simulink model "control_scenario2"  (Simulink 8.9)
settings: Solver=FixedStepAuto  StartTime=0.0  StopTime=20  MaxStep=0.01  RelTol=1e-4  EnableMultiTasking=on
undefined symbols (not defined in the file or in its folder): sigbuilder_block
libraries: fuzblock x1
settings Model: LogicAnalyzerSignalOrdering=6b2a1942-3d28-4729-8a02-0566cc64ad92,33d7c2ba-298a-487f-a15a-bbe0029d2366,768ba1eb-50de-46f7-9be9-bebabd7bf970,4ab0f0e9-8454-41f6-a2d7-33861cd3e8d9  SuppressorTable=22 serialization::archive 11 0 6 0 0 0 11 0  Creator=root  LastModifiedBy=root
settings Model: LogicAnalyzerGraphicalSettings=|
  | {
  |   "cursors" : {
  |     "activeCursor" : 0,
  |     "lockedCursors" : [
  | 
  |     ],
  |     "startingCursor" : 0,
  |     "times" : [
  |       0
  |     ]
  |   },
  |   "global" : {
  |   },
  |   "panels" : [
  |     {
  |       "height" : 100,
  |       "startingTrace" : 0,
  |       "traces" : [
  |         {
  |           "signalId" : "33d7c2ba-298a-487f-a15a-bbe0029d2366",
  |           "type" : "wave"
  |         },
  |         {
  |           "signalId" : "768ba1eb-50de-46f7-9be9-bebabd7bf970",
  |           "type" : "wave"
  |         },
  |         {
  |           "signalId" : "4ab0f0e9-8454-41f6-a2d7-33861cd3e8d9",
  |           "type" : "wave"
  |         },
  |         {
  |           "signalId" : "6b2a1942-3d28-4729-8a02-0566cc64ad92",
  |           "type" : "wave"
  |         }
  |       ],
  |       "yOffset" : 0
  |     }
  |   ],
  |   "timeAxis" : {
  |     "displayUnits" : "",
  |     "pixelsPerSecond" : 293
  |   }
  | }
settings DataIOCC: SaveFormat=Dataset  SignalLoggingSaveFormat=Dataset  SaveOutput=off  SaveTime=off
settings OptimizationCC: ExpressionDepthLimit=2147483647  LifeSpan=1
settings DebuggingCC: AllowSymbolicDim=off
settings HardwareCC: ProdBitPerPointer=64  ProdBitPerSizeT=64  ProdBitPerPtrDiffT=64  ProdLargestAtomicFloat=Float  ProdIntDivRoundTo=Zero  ProdEndianess=LittleEndian  ProdWordSize=64  ProdHWDeviceType=Intel->x86-64 (Windows64)
settings ModelReferenceCC: PropagateSignalLabelsOutOfModel=on
settings ConfigComp: CovMetricSettings=dwe  CovHtmlReporting=off  CovSaveCumulativeToWorkspaceVar=off  CovSaveSingleToWorkspaceVar=off  CovExternalEMLEnable=on

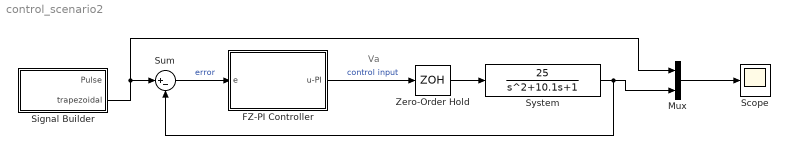
== system control_scenario2 ==
  note: Va
  FZ-PI Controller : Subsystem
  Mux : Mux  Inputs=2
  Scope : Scope
  Signal Builder : Subsystem  Tag=STV Subsys  LoadFcn=sigbuilder_block('load');  StartFcn=sigbuilder_block('start');  StopFcn=sigbuilder_block('stop');  ClipboardFcn=sigbuilder_block('clipboard');  mask(Sigbuilder block){tuvar=[0:10]}
      mask help: Simulink:masks:SigbuilderBlock_MD
      mask init:
      | if ~strcmp(get_param(bdroot(gcbh),'SimulationStatus'),'stopped') tuvar = sigbuilder_block('maskInit'); end
      settings: CopyFcn=sigbuilder_block('copy');  DeleteFcn=sigbuilder_block('delete');  ModelCloseFcn=sigbuilder_block('modelClose');  PreSaveFcn=sigbuilder_block('preSave');  PauseFcn=sigbuilder_block('pause');  ContinueFcn=sigbuilder_block('continue');  NameChangeFcn=sigbuilder_block('namechange');  OpenFcn=sigbuilder_block('open',[136.5 202.5 558 422.25 ]);  CloseFcn=sigbuilder_block('close');
      mask Display: plot(0, 0, 100, 100,[2, 2, 32, 32, 2], [68, 8, 8, 68, 68],[32, 2], [38, 38], [32, 19, 2],[53, 60, 44], [32, 17, 17, 2],[16, 16, 31, 31]);txt = getActiveGroup(gcbh);text(2, 100, txt,'verticalAlignment', 'top');
  Sum : Sum  Inputs=|+-
  System : TransferFcn  Numerator=[25]  Denominator=[1 10.1 1]
  Zero-Order Hold : ZeroOrderHold  SampleTime=0.01
  wires:
  Sum/1 -> FZ-PI Controller/1(e)  "error"
  FZ-PI Controller/1(u-PI) -> Zero-Order Hold/1  "control input"
  Zero-Order Hold/1 -> System/1
  System/1 -> Sum/2, Mux/2
  Mux/1 -> Scope/1
  Signal Builder/2(trapezoidal) -> Mux/1, Sum/1

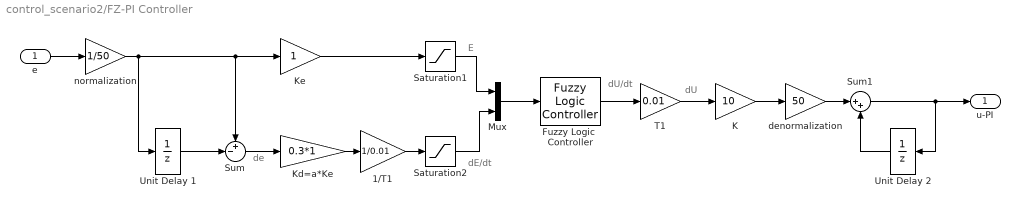
== system control_scenario2/FZ-PI Controller ==
  note: E
  note: de
  note: dE/dt
  note: dU/dt
  note: dU
  e : Inport
  1/T1 : Gain  Gain=1/0.01
  Fuzzy Logic  Controller : fuzblock/Fuzzy Logic  Controller  fis='fis.fis'
  K : Gain  Gain=10
  Kd=a*Ke : Gain  Gain=0.3*1
  Mux : Mux  Inputs=2
  Saturation1 : Saturate  UpperLimit=1  LowerLimit=-1
  Saturation2 : Saturate  UpperLimit=1  LowerLimit=-1
  Sum : Sum  Inputs=+-|
  Sum1 : Sum  Inputs=|++
  "T1 " : Gain  Gain=0.01
  Unit Delay 1 : UnitDelay  SampleTime=0.01
  Unit Delay 2 : UnitDelay  SampleTime=0.01
  denormalization : Gain  Gain=50
  normalization : Gain  Gain=1/50
  Κe : Gain
  u-PI : Outport
  wires:
  e/1 -> normalization/1
  normalization/1 -> Unit Delay 1/1, Sum/1, Κe/1
  Unit Delay 1/1 -> Sum/2
  Sum/1 -> Kd=a*Ke/1
  Kd=a*Ke/1 -> 1/T1/1
  Κe/1 -> Saturation1/1
  1/T1/1 -> Saturation2/1
  Saturation1/1 -> Mux/1
  Saturation2/1 -> Mux/2
  Mux/1 -> Fuzzy Logic  Controller/1
  Fuzzy Logic  Controller/1 -> "T1 "/1
  "T1 "/1 -> K/1
  K/1 -> denormalization/1
  denormalization/1 -> Sum1/1
  Sum1/1 -> u-PI/1, Unit Delay 2/1
  Unit Delay 2/1 -> Sum1/2

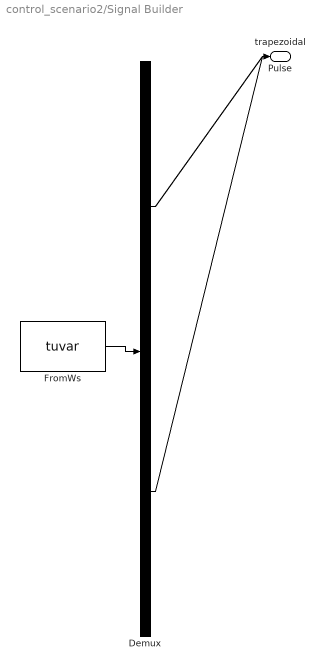
== system control_scenario2/Signal Builder ==
  Demux : Demux  Tag=STV Demux  Outputs=2
  FromWs : FromWorkspace  Tag=STV FromWs  VariableName=tuvar  SampleTime=0  SigBuilderData=DataTag0  VnvData=DataTag1
      SigBuilderData=|
      | common.afterFinalStr = 'Extrapolate'
      | common.sampleTime = 0
      | dataSet.timeRange = [0 15]
      | dataSet.name = 'Group 1'
      | sbobj.Groups.Name = 'Group 1'
      | sbobj.Groups.Signals(1).Name = 'Pulse'
      | sbobj.Groups.Signals(1).XData = [0 5 5 10 10 15]
      | sbobj.Groups.Signals(1).YData = [50 50 20 20 40 40]
      | sbobj.Groups.Signals(2).Name = 'trapezoidal'
      | sbobj.Groups.Signals(2).XData = [0 5 10 15]
      | sbobj.Groups.Signals(2).YData = [0 50 50 25]
      | sbobj.Groups.TimeRange = [0 15]
  Pulse : Outport  Tag=STV Outport
  trapezoidal : Outport  Tag=STV Outport  Port=2
  wires:
  FromWs/1 -> Demux/1
  Demux/1 -> Pulse/1
  Demux/2 -> trapezoidal/1
